simulink subsystem "MOTOR_"  (R2023a)
settings: Solver=VariableStepAuto  StartTime=0.0  StopTime=10.0  RelTol=1e-3
settings Model: Creator=hidra  LastModifiedBy=hidra

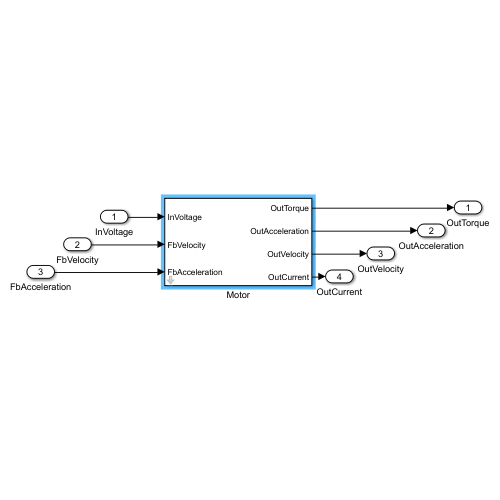
[thumbnail: Simulink's stored preview of the top-level diagram]
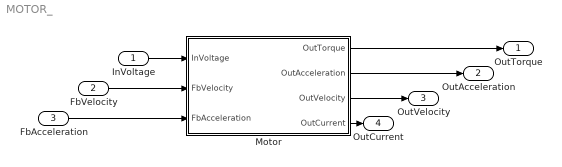
== system MOTOR_ ==
  InVoltage : Inport
  FbVelocity : Inport  Port=2
  FbAcceleration : Inport  Port=3
  Motor : Subsystem  mask{R=10, L=0.000350, k_vel=10, k_mom=0.016, J=0.0000005, k_vask=0.5}
      mask prompts: R "Активное сопротивление якоря, Ом"; L "Индуктивность якоря, Гн"; k_vel "Коэф. скорости двигателя, об/сек"; k_mom "Коэф. момента двигателя, Н*м/А"; J "Момент инерции, кг*м^2"; k_vask "Коэф. вязкого трения двигателя"
  OutTorque : Outport
  OutAcceleration : Outport  Port=2
  OutVelocity : Outport  Port=3
  OutCurrent : Outport  Port=4
  wires:
  Motor/1(OutTorque) -> OutTorque/1
  Motor/2(OutAcceleration) -> OutAcceleration/1
  Motor/3(OutVelocity) -> OutVelocity/1
  Motor/4(OutCurrent) -> OutCurrent/1
  InVoltage/1 -> Motor/1(InVoltage)
  FbVelocity/1 -> Motor/2(FbVelocity)
  FbAcceleration/1 -> Motor/3(FbAcceleration)

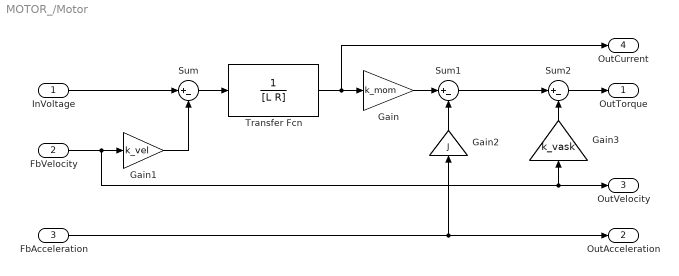
== system MOTOR_/Motor ==
  InVoltage : Inport
  FbVelocity : Inport  Port=2
  FbAcceleration : Inport  Port=3
  Gain : Gain  Gain=k_mom
  Gain1 : Gain  Gain=k_vel
  Gain2 : Gain  Gain=J
  Gain3 : Gain  Gain=k_vask
  Sum : Sum  Inputs=|+-
  Sum1 : Sum  Inputs=|+-
  Sum2 : Sum  Inputs=|+-
  Transfer Fcn : TransferFcn  Denominator=[L R]
  OutTorque : Outport
  OutAcceleration : Outport  Port=2
  OutVelocity : Outport  Port=3
  OutCurrent : Outport  Port=4
  wires:
  InVoltage/1 -> Sum/1
  Sum/1 -> Transfer Fcn/1
  Transfer Fcn/1 -> Gain/1, OutCurrent/1
  FbVelocity/1 -> OutVelocity/1, Gain3/1, Gain1/1
  Gain1/1 -> Sum/2
  FbAcceleration/1 -> OutAcceleration/1, Gain2/1
  Gain/1 -> Sum1/1
  Gain2/1 -> Sum1/2
  Sum1/1 -> Sum2/1
  Sum2/1 -> OutTorque/1
  Gain3/1 -> Sum2/2
